simulink model "PIDdiscret_01"  (Simulink 8.5)
settings: Solver=ode3  StartTime=0.0  StopTime=7  FixedStep=0.1  RelTol=1e-3
values from neighbouring files (symbols this model uses):
  K = (y_real(end) - y_real(1))/(input.signals.values(end) - 0)    [ctr.m]
  L = 1.5*(t1_28 - (t2_63/3))    [ctr.m]
  T = 1.5*(t2_63 - t1_28)    [ctr.m]
settings Model: Creator=guima  LastModifiedBy=guima
settings DataIOCC: SignalLoggingSaveFormat=Dataset
settings OptimizationCC: ExpressionDepthLimit=128
settings DebuggingCC: UnderspecifiedInitializationDetection=Simplified  MergeDetectMultiDrivingBlocksExec=error  FcnCallInpInsideContextMsg=EnableAllAsError  StateNameClashWarn=none
settings GRTTargetCC: CombineOutputUpdateFcns=on  GRTInterface=off

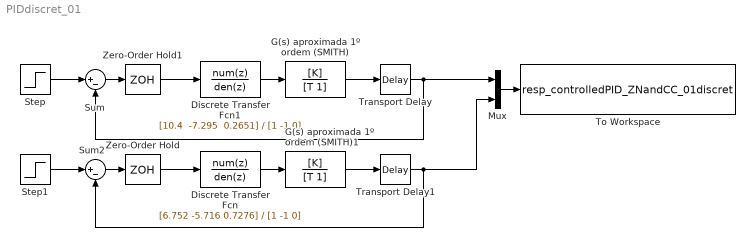
== system PIDdiscret_01 ==
  Discrete Transfer Fcn : DiscreteTransferFcn  Numerator=[6.752 -5.716 0.7276]  Denominator=[1 -1 0]  SampleTime=0.1
  Discrete Transfer Fcn1 : DiscreteTransferFcn  Numerator="[10.4  -7.295  0.2651]"  Denominator=[1 -1 0]  SampleTime=0.1
  G(s) aproximada 1º ordem (SMITH) : TransferFcn  Numerator=[K]  Denominator=[T 1]
  G(s) aproximada 1º ordem (SMITH)1 : TransferFcn  Numerator=[K]  Denominator=[T 1]
  Mux : Mux  Inputs=2
  Step : Step  Time=0  SampleTime=0
  Step1 : Step  Time=0  SampleTime=0
  Sum : Sum  Inputs=|+-
  Sum2 : Sum  Inputs=|+-
  To Workspace : ToWorkspace  VariableName=resp_controlledPID_ZNandCC_01discret  SaveFormat=Structure With Time  SampleTime=-1
  Transport Delay : TransportDelay  DelayTime=L
  Transport Delay1 : TransportDelay  DelayTime=L
  Zero-Order Hold : ZeroOrderHold  SampleTime=0.1
  Zero-Order Hold1 : ZeroOrderHold  SampleTime=0.1
  wires:
  Step/1 -> Sum/1
  Sum/1 -> Zero-Order Hold1/1
  Discrete Transfer Fcn1/1 -> G(s) aproximada 1º ordem (SMITH)/1
  G(s) aproximada 1º ordem (SMITH)/1 -> Transport Delay/1
  Transport Delay/1 -> Mux/1, Sum/2
  Step1/1 -> Sum2/1
  G(s) aproximada 1º ordem (SMITH)1/1 -> Transport Delay1/1
  Transport Delay1/1 -> Sum2/2, Mux/2
  Mux/1 -> To Workspace/1
  Sum2/1 -> Zero-Order Hold/1
  Discrete Transfer Fcn/1 -> G(s) aproximada 1º ordem (SMITH)1/1
  Zero-Order Hold/1 -> Discrete Transfer Fcn/1
  Zero-Order Hold1/1 -> Discrete Transfer Fcn1/1
